simulink model "single_engine_test"  (R2018b)
settings: Solver=FixedStepAuto  StartTime=0.0  StopTime=0.02  FixedStep=0.0001  RelTol=1e-3
settings Model: Creator=Paweł Tymiński  LastModifiedBy=Paweł Tymiński

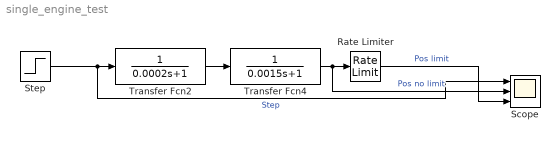
== system single_engine_test ==
  Rate Limiter : RateLimiter  RisingSlewLimit=58.6  FallingSlewLimit=-58.6  SampleTimeMode=inherited
  Scope : Scope  NumInputPorts=3
  Step : Step  Time=0  SampleTime=0
  Transfer Fcn2 : TransferFcn  Denominator=[0.0002 1]
  Transfer Fcn4 : TransferFcn  Denominator=[0.0015 1]
  wires:
  Rate Limiter/1 -> Scope/3  "Pos limit"
  Transfer Fcn4/1 -> Scope/2, Rate Limiter/1  "Pos no limit"
  Step/1 -> Scope/1, Transfer Fcn2/1  "Step"
  Transfer Fcn2/1 -> Transfer Fcn4/1
